simulink model "LKAS_AutoSave_DF_20220215_0920"  (R2018b)
settings: Solver=FixedStepDiscrete  StartTime=0.0  StopTime=10.0  FixedStep=0.01  RelTol=1e-3
InitFcn:
  | tmpVer = ver('MATLAB');
  | tmpVer = str2num(tmpVer.Version);
  | % -------------------------------------------------------------------
  | %  MATLAB file generated by Simulink.saveVars on 21-Nov-2019 10:06:14
  | %  MATLAB version: 7.13.0.564 (R2011b)
  | % -------------------------------------------------------------------
  | 
  | 
  | SInt16 = Simulink.AliasType;
  | SInt16.Description = 'Num';
  | if (tmpVer > 7.11)
  | 	SInt16.DataScope = 'Auto';
  | end
  | SInt16.HeaderFile = 'Rte_Type.h';
  | SInt16.BaseType = 'int16';
  | 
  | SInt32 = Simulink.AliasType;
  | SInt32.Description = 'Num';
  | if (tmpVer > 7.11)
  | 	SInt32.DataScope = 'Auto';
  | end
  | SInt32.HeaderFile = 'Rte_Type.h';
  | SInt32.BaseType = 'int32';
  | 
  | SInt8 = Simulink.AliasType;
  | SInt8.Description = 'Num';
  | if (tmpVer > 7.11)
  | 	SInt8.DataScope = 'Auto';
  | end
  | SInt8.HeaderFile = 'Rte_Type.h';
  | SInt8.BaseType = 'int8';
  | 
  | T_A_m2_1024_1_u32 = Simulink.NumericType;
  | T_A_m2_1024_1_u32.Description = 'm2 (square meters  (m2))';
  | if (tmpVer > 7.11)
  | 	T_A_m2_1024_1_u32.DataScope = 'Auto';
  | end
  | T_A_m2_1024_1_u32.HeaderFile = 'Rte_Type.h';
  | T_A_m2_1024_1_u32.DataTypeMode = 'Fixed-point: slope and bias scaling';
  | T_A_m2_1024_1_u32.SignednessBool = false;
  | T_A_m2_1024_1_u32.WordLength = 32;
  | T_A_m2_1024_1_u32.FixedExponent = -10;
  | T_A_m2_1024_1_u32.SlopeAdjustmentFactor = 1;
  | T_A_m2_1024_1_u32.Bias = 0;
  | T_A_m2_1024_1_u32.DataTypeOverride = 'Inherit';
  | T_A_m2_1024_1_u32.IsAlias = true;
  | 
  | T_A_m2_65536_1_u16 = Simulink.NumericType;
  | T_A_m2_65536_1_u16.Description = 'm2 (square meters  (m2))';
  | if (tmpVer > 7.11)
  | 	T_A_m2_65536_1_u16.DataScope = 'Auto';
  | end
  | T_A_m2_65536_1_u16.HeaderFile = 'Rte_Type.h';
  | T_A_m2_65536_1_u16.DataTypeMode = 'Fixed-point: slope and bias scaling';
  | T_A_m2_65536_1_u16.SignednessBool = false;
  | T_A_m2_65536_1_u16.WordLength = 16;
  | T_A_m2_65536_1_u16.FixedExponent = -16;
  | T_A_m2_65536_1_u16.SlopeAdjustmentFactor = 1;
  | T_A_m2_65536_1_u16.Bias = 0;
  | T_A_m2_65536_1_u16.DataTypeOverride = 'Inherit';
  | ... (+4647 lines)
StopFcn:
  | clear  T_A_m2_1024_1_u32 T_A_m2_65536_1_u16 T_A_m2_Float32 T_A_mm2_10_1_u16 T_A_mm2_4_1_s16 T_A_mm2_Float32 T_Cnt_Num_10_1_u32 T_Cnt_Num_1_1_s16 T_Cnt_Num_1_1_s32 T_Cnt_Num_1_1_s8 T_Cnt_Num_1_1_u16 T_Cnt_Num_1_1_u32 T_Cnt_Num_1_1_u8 T_E_J_1_1_s32 T_E_J_Float32 T_E_kJ_128_1_s32 T_E_kJ_Float32 T_E_kwh_10_1_u16 T_E_kwh_Float32 T_Epl_kwhpkm_100_1_u16 T_Epl_kwhpkm_Float32 T_F_N_1_1_s16 T_F_N_Float32 T_I_A_1000_1_u16 T_I_A_1048576_1_s32 T_I_A_2048_1_s16 T_I_A_32_1_s16 T_I_A_Float32 T_I_mA_1_1_s16 T_I_mA_32768_128_s16 T_I_mA_Float32 T_J_kgpm2_128_1_u16 T_J_kgpm2_Float32 T_K_NA_1000_1_s16 T_K_NA_100_1_s16 T_K_NA_100_1_u16 T_K_NA_1024_1_s16 T_K_NA_1024_1_u16 T_K_NA_128_1_s16 T_K_NA_128_1_u16 T_K_NA_128_1_u8 T_K_NA_16777216_1_u32 T_K_NA_16_1_s16 T_K_NA_16_1_u16 T_K_NA_16_1_u8 T_K_NA_1_16_u16 T_K_NA_1_1_s16 T_K_NA_1_1_u16 T_K_NA_1_1_u8 T_K_NA_32768_1_s16 T_K_NA_32768_1_u16 T_K_NA_32_1_s8 T_K_NA_4096_1_u16 T_K_NA_4194304_1_s32 T_K_NA_4194304_1_u16 T_K_NA_65536_1_s32 T_K_NA_65536_1_u16 T_K_NA_8192_1_s16 T_K_NA_8_1_s16 T_K_NA_Float32 T_M_Nm_16_1_s16 T_M_Nm_1_1_s16 T_M_Nm_32768_1_s16 T_M_Nm_32_1_s16 T_M_Nm_4_1_s16 T_M_Nm_512_1_s16 T_M_Nm_Float32 T_P_W_1_4_s16 T_P_W_1_8_s16 T_P_W_Float32 T_P_kW_128_1_s16 T_P_kW_1_8_s16 T_P_kW_8_1_s32 T_P_kW_Float32 T_Pct_pct_1024_1_s32 T_Pct_pct_1024_1_u32 T_Pct_pct_10_1_s16 T_Pct_pct_10_1_u32 T_Pct_pct_128_100_s8 T_Pct_pct_1_1_s16 T_Pct_pct_1_4_u8 T_Pct_pct_255_100_u16 T_Pct_pct_255_100_u8 T_Pct_pct_256_1_s16 T_Pct_pct_256_1_u16 T_Pct_pct_65535_100_u16 T_Pct_pct_Float32 T_R_ohm_1024_1_s16 T_R_ohm_32_1_s16 T_R_ohm_Float32 T_TK_K_16_1_s16 T_TK_K_Float32 T_T_degC_10_400_1_u16 T_T_degC_16_1_s16 T_T_degC_1_40_1_u8 T_T_degC_2_80_1_u8 T_T_degC_Float32 T_U_V_1000_1_u16 T_U_V_10_1_u8 T_U_V_200_1_u8 T_U_V_32_1_s16 T_U_V_4096_1_s16 T_U_V_512_1_s16 T_U_V_65535_8_u16 T_U_V_8192_1_u16 T_U_V_Float32 T_U_mV_1_1_s16 T_U_mV_256_20_u16 T_U_mV_Float32 T_V_l_256_1_s16 T_V_l_4096_1_s16 T_V_l_64_1_s16 T_V_l_65535_100_u16 T_V_l_Float32 T_V_ml_128_1_s16 T_V_ml_1_1_s16 T_V_ml_32768_1_s16 T_V_ml_Float32 T_V_ul_32_1_u16 T_V_ul_Float32 T_Vpl_clpkm_512_1_u16 T_Vpl_clpkm_Float32 T_a_kphps_16_1_s16 T_a_kphps_Float32 T_a_mps2_128_1_s16 T_a_mps2_Float32 T_c_MJpkg_256_1_s16 T_c_MJpkg_Float32 T_c_kJpgpK_1024_1_s16 T_c_kJpgpK_Float32 T_c_kJpkgpK_128_1_u16 T_c_kJpkgpK_Float32 T_chrg_Ah_1_1_s16 T_chrg_Ah_1_1_u16 T_chrg_Ah_1_1_u8 T_chrg_Ah_256_1_u16 T_chrg_Ah_4194304_1_s32 T_chrg_Ah_512_1_u16 T_chrg_Ah_8_1_u16 T_chrg_Ah_Float32 T_cmp_NA_100_1_s16 T_cmp_NA_128_1_s16 T_cmp_NA_16_1_s16 T_cmp_NA_32768_1_u16 T_cmp_NA_Float32 T_d2n_rpmps2_4_1_s16 T_d2n_rpmps2_Float32 T_dPct_pctps_16_1_s16 T_dPct_pctps_256_1_s16 T_dPct_pctps_Float32 T_dT_degCps_128_1_s16 T_dT_degCps_Float32 T_dV_lph_1_1_s16 T_dV_lph_Float32 T_dV_lpm_128_1_s16 T_dV_lpm_32_1_s16 T_dV_lpm_Float32 T_dV_lps_1024_1_u16 T_dV_lps_4_1_u16 T_dV_lps_Float32 T_dV_mlps_1024_1_s16 T_dV_mlps_Float32 T_d_BitField16 T_dm_gps_128_1_s16 T_dm_gps_128_1_u16 T_dm_gps_256_1_u16 T_dm_gps_Float32 T_dm_mgps_1_1_s16 T_dm_mgps_Float32 T_dn_rpmps_1_1_s16 T_dn_rpmps_2_1_s16 T_dn_rpmps_Float32 T_dp_Paps_1_1_s16 T_dp_Paps_Float32 T_dp_kPaps_1_1_s16 T_dp_kPaps_8_1_s16 T_dp_kPaps_Float32 T_dphi_degps_128_1_s16 T_dphi_degps_8_1_s16 T_dphi_degps_Float32 T_dr_ps_256_1_s16 T_dr_ps_Float32 T_drho_mgplps_1_2_s16 T_drho_mgplps_Float32 T_e_NA_1_1_u8 T_f_Hz_1_1_u16 T_f_Hz_1_1_u32 T_f_Hz_64_1_u16 T_f_Hz_8_1_s16 T_f_Hz_Float32 T_g_BitField32 T_l_km_16_1_s16 T_l_km_1_1_u16 T_l_km_1_1_u32 T_l_km_Float32 T_l_m_1024_1_s16 T_l_m_16_1_s16 T_l_m_1_1_u32 T_l_m_Float32 T_l_mm_16_1_s16 T_l_mm_1_1_u16 T_l_mm_4096_1_s16 T_l_mm_4_1_u8 T_l_mm_64_1_s16 T_l_mm_Float32 T_m_g_1_1_s16 T_m_g_2048_1_s16 T_m_g_32_1_u16 T_m_g_Float32 T_m_kg_1024_1_s16 T_m_kg_1_1_s16 T_m_kg_1_1_u32 T_m_kg_Float32 T_m_mg_128_1_s16 T_m_mg_32_1_s16 T_m_mg_Float32 T_n_rpm_1_1_s16 T_n_rpm_1_25_u8 T_n_rpm_256_50_u16 T_n_rpm_2_25_u8 T_n_rpm_4_1_u16 T_n_rpm_Float32 T_p_MPa_64_1_s16 T_p_MPa_Float32 T_p_Pa_1_1_s16 T_p_Pa_Float32 T_p_kPa_1_10_u16 T_p_kPa_1_1_s16 T_p_kPa_1_1_u8 T_p_kPa_256_1_u16 T_p_kPa_32_1_u16 T_p_kPa_64_1_s16 T_p_kPa_Float32 T_phi_deg_100_1_s16 T_phi_deg_1024_1_s16 T_phi_deg_128_1_s16 T_phi_deg_1_1_u8 T_phi_deg_256_1_s16 T_phi_deg_2_1_s8 T_phi_deg_32_1_s16 T_phi_deg_512_6_s32 T_phi_deg_Float32 T_phi_rad_2048_1_s16 T_phi_rad_Float32 T_r_NA_1024_1_s16 T_r_NA_1024_1_u16 T_r_NA_16384_1_s16 T_r_NA_16_1_s16 T_r_NA_256_1_s8 T_r_NA_256_1_u16 T_r_NA_32768_1_u16 T_r_NA_32_1_u16 T_r_NA_4096_1_s16 T_r_NA_65535_2_u16 T_r_NA_8192_1_u16 T_r_NA_Float32 T_rho_gpl_8192_1_s16 T_rho_gpl_Float32 T_rho_kgpm3_16_1_s16 T_rho_kgpm3_Float32 T_rho_mgpl_1_1_s16 T_rho_mgpl_64_1_s16 T_rho_mgpl_Float32 T_t_hour_1_1_s16 T_t_hour_Float32 T_t_m_1_1_u16 T_t_m_Float32 T_t_ms_1_1_s16 T_t_ms_1_1_u16 T_t_ms_1_1_u32 T_t_ms_4096_1_s16 T_t_ms_64_1_s16 T_t_ms_Float32 T_t_s_1000_1_s16 T_t_s_100_1_s16 T_t_s_10_1_s16 T_t_s_10_1_u16 T_t_s_1_1_s16 T_t_s_1_1_u16 T_t_s_1_1_u32 T_t_s_Float32 T_t_us_10_1_u32 T_t_us_1_1_s16 T_t_us_1_1_u32 T_t_us_1_4_u16 T_t_us_Float32 T_v_kph_1_1_u8 T_v_kph_64_1_s16 T_v_kph_64_1_u16 T_v_kph_Float32 T_v_mps_256_1_s16 T_v_mps_Float32 T_w_radps_32_1_s16 T_w_radps_Float32 T_y_BitField8 T_y_BitFieldDiagProgress T_y_BitFieldDiagStatus T_y_NA_1_1_u8 SInt16 SInt32 SInt8 T_BOOLEAN UInt16 UInt32 UInt8 s16 s32 s8 u16 u32 u8
model workspace (MAT data in the model file):
  MCOS : class17 (value not decoded)
  MCOS : class17 (value not decoded)
  MCOS : class17 (value not decoded)
  MCOS : class17 (value not decoded)
  MCOS : class17 (value not decoded)
  MCOS : class17 (value not decoded)
  MCOS : class17 (value not decoded)
  MCOS : class17 (value not decoded)
  MCOS : class17 (value not decoded)
  MCOS : class17 (value not decoded)
  MCOS : class17 (value not decoded)
  MCOS : class17 (value not decoded)
  MCOS : class17 (value not decoded)
  MCOS : class17 (value not decoded)
  MCOS : class17 (value not decoded)
  MCOS : class17 (value not decoded)
  MCOS : class17 (value not decoded)
  MCOS : class17 (value not decoded)
  MCOS : class17 (value not decoded)
  MCOS : class17 (value not decoded)
  MCOS : class17 (value not decoded)
  MCOS : class17 (value not decoded)
  MCOS : class17 (value not decoded)
  MCOS : class17 (value not decoded)
  MCOS : class17 (value not decoded)
  MCOS : class17 (value not decoded)
  MCOS : class17 (value not decoded)
  MCOS : class17 (value not decoded)
  MCOS : class17 (value not decoded)
  MCOS : class17 (value not decoded)
  MCOS : class17 (value not decoded)
  MCOS : class17 (value not decoded)
  MCOS : class17 (value not decoded)
  MCOS : class17 (value not decoded)
  MCOS : class17 (value not decoded)
  MCOS : class17 (value not decoded)
  MCOS : class17 (value not decoded)
  MCOS : class17 (value not decoded)
  MCOS : class17 (value not decoded)
  MCOS : class17 (value not decoded)
  MCOS : class17 (value not decoded)
  MCOS : class17 (value not decoded)
  MCOS : class17 (value not decoded)
  MCOS : class17 (value not decoded)
  MCOS : class17 (value not decoded)
  MCOS : class17 (value not decoded)
  MCOS : class17 (value not decoded)
  MCOS : class17 (value not decoded)
  MCOS : class17 (value not decoded)
  MCOS : class17 (value not decoded)
  MCOS : class17 (value not decoded)
  MCOS : class17 (value not decoded)
  MCOS : class17 (value not decoded)
  MCOS : class17 (value not decoded)
  MCOS : class17 (value not decoded)
  MCOS : class17 (value not decoded)
  MCOS : class17 (value not decoded)
  MCOS : class17 (value not decoded)
  MCOS : class17 (value not decoded)
  MCOS : class17 (value not decoded)
  MCOS : class17 (value not decoded)
  MCOS : class17 (value not decoded)
  MCOS : class17 (value not decoded)
  MCOS : class17 (value not decoded)
  MCOS : class17 (value not decoded)
  MCOS : class17 (value not decoded)
  MCOS : class17 (value not decoded)
  MCOS : class17 (value not decoded)
  MCOS : class17 (value not decoded)
  MCOS : class17 (value not decoded)
  MCOS : class17 (value not decoded)
  MCOS : class17 (value not decoded)
  MCOS : class17 (value not decoded)
  MCOS : class17 (value not decoded)
  MCOS : class17 (value not decoded)
  MCOS : class17 (value not decoded)
  MCOS : class17 (value not decoded)
  MCOS : class17 (value not decoded)
  MCOS : class17 (value not decoded)
  MCOS : class17 (value not decoded)
  MCOS : class17 (value not decoded)
  MCOS : class17 (value not decoded)
  MCOS : class17 (value not decoded)
  MCOS : class17 (value not decoded)
  MCOS : class17 (value not decoded)
  MCOS : class17 (value not decoded)
  MCOS : class17 (value not decoded)
  MCOS : class17 (value not decoded)
  MCOS : class17 (value not decoded)
  MCOS : class17 (value not decoded)
  MCOS : class17 (value not decoded)
  MCOS : class17 (value not decoded)
  MCOS : class17 (value not decoded)
  MCOS : class17 (value not decoded)
  MCOS : class17 (value not decoded)
  MCOS : class17 (value not decoded)
  MCOS : class17 (value not decoded)
  MCOS : class17 (value not decoded)
  MCOS : class17 (value not decoded)
  MCOS : class17 (value not decoded)
  MCOS : class17 (value not decoded)
  MCOS : class17 (value not decoded)
undefined symbols (not defined in the file): LKA_CarWidth, LKA_SampleTime, LKA_StrRatio_C, LKA_Veh2CamL_C, LKA_Veh2CamW_C, LKA_WhlBaseL_C, LL_CompHdAg_C, LL_CompSWA_C, LL_CrvtPrvwT_C, LL_DesDvt_C, LL_DvtComp_C, LL_DvtPrvwT_C, LL_DvtSpdDet_vDvtSpdMin_C, LL_HandsOff_ExitTime, LL_HandsOff_TextTime, LL_HandsOff_WarnTime, LL_HdAgExT_C, LL_HdAgPrvwT_C, LL_LAccMax_C, LL_LAccRMax_C, LL_LDW_EarliestWarnLine_C, LL_LDW_LatestWarnLine_C, LL_LDWS_SUPPRESS_HEADING, LL_LFClb_TFC_FfCtlRatio_C, LL_LFClb_TFC_KdBalance_C, LL_LFClb_TFC_KdMaxSWA_C, LL_LFClb_TFC_KdV1_C, LL_LFClb_TFC_KdV2_C, LL_LFClb_TFC_KdVehSpdLwr_C, LL_LFClb_TFC_KdVehSpdUpr_C, LL_LFClb_TFC_Ki_C, LL_LFClb_TFC_KiMaxSWA_C, LL_LFClb_TFC_Kp_C, LL_LFClb_TFC_KpKlat_C, LL_LFClb_TFC_KpV1_C, LL_LFClb_TFC_KpV2_C, LL_LFClb_TFC_KpVehSpdLwr_C, LL_LFClb_TFC_KpVehSpdUpr_C, LL_LFClb_TFC_PrvwT_C, LL_LKA_EarliestWarnLine_C, LL_LKA_LatestWarnLine_C, LL_LKAExPrcs_ExitC0Dvt, LL_LKAExPrcs_ExitC0Swt, LL_LKAExPrcs_tiExitTime1, LL_LKAExPrcs_tiExitTime2, LL_LKAExPrcs_tiExitTime3, LL_LKAS_OUT_OF_CONTROL_LAT_VEL, LL_LKAS_OUT_OF_CONTROL_TTLC, LL_LKASWASyn_M0, LL_LKASWASyn_M1, LL_LKASWASyn_M2, LL_LKASWASyn_M3K, LL_LKASWASyn_SWAaddMax, LL_LKASWASyn_T2, LL_LKASWASyn_tiTrqSwaRtTime, LL_LKASWASyn_tiTrqSwaTime, LL_LKASWASyn_TrqMax, LL_LKASWASyn_TrqSwaAddSwt, LL_LKASWASyn_TrqSwaRateDiff, LL_LSpdCompT_C ... (+43)
libraries: simulink x136, canmsglib x8, dspstat3 x3, simulink_extras x1
(part 4 of 20)

== system LKAS_AutoSave_DF_20220215_0920/LKAS/Monitor ==
  CAN Pack : canmsglib/CAN Pack  MsgList=(none)  MsgName=CAN Msg  MsgIDType=Standard (11-bit identifier)  MsgIdentifier=1  MsgLength=8  SignalInfo=Signal1$8$16$2$2$1$0$0.01$0$-Inf$Inf$#Signal2$24$16$2$2$1$0$0.01$0$-Inf$Inf$#Signal3$40$16$2$2$1$0$0.01$0$-Inf$Inf$#Signal4$56$16$2$2$1$0$0.01$0$-Inf$Inf$#  NSignals=4  StartBits=str2num('[int32(8);int32(24);int32(40);int32(56)]')  SignalSizes=str2num('[int32(16);int32(16);int32(16);int32(16)]')  ByteOrders=str2num('[int32(2);int32(2);int32(2);int32(2)]')  DataTypes=str2num('[int32(2);int32(2);int32(2);int32(2)]')  MultiplexTypes=str2num('[int32(1);int32(1);int32(1);int32(1)]')  MultiplexValues=str2num('[double(0);double(0);double(0);double(0)]')  Factors=str2num('[double(0.01);double(0.01);double(0.01);double(0.01)]')  Offsets=str2num('[double(0);double(0);double(0);double(0)]')  Minimums=str2num('[double(-Inf);double(-Inf);double(-Inf);double(-Inf)]')  Maximums=str2num('[double(Inf);double(Inf);double(Inf);double(Inf)]')  Remote=off  ApplyMinMax=off  BusOutput=on
      settings: SourceProductName=Simulink Real-Time  SourceProductBaseCode=XP  DataFormat=manually specified signals
  CAN Pack1 : canmsglib/CAN Pack  MsgList=(none)  MsgName=CAN Msg  MsgIDType=Standard (11-bit identifier)  MsgIdentifier=2  MsgLength=8  SignalInfo=Signal1$8$16$2$2$1$0$0.01$0$-Inf$Inf$#Signal2$24$16$2$2$1$0$0.01$0$-Inf$Inf$#Signal3$40$16$2$2$1$0$0.01$0$-Inf$Inf$#Signal4$56$16$2$2$1$0$0.01$0$-Inf$Inf$#  NSignals=4  StartBits=str2num('[int32(8);int32(24);int32(40);int32(56)]')  SignalSizes=str2num('[int32(16);int32(16);int32(16);int32(16)]')  ByteOrders=str2num('[int32(2);int32(2);int32(2);int32(2)]')  DataTypes=str2num('[int32(2);int32(2);int32(2);int32(2)]')  MultiplexTypes=str2num('[int32(1);int32(1);int32(1);int32(1)]')  MultiplexValues=str2num('[double(0);double(0);double(0);double(0)]')  Factors=str2num('[double(0.01);double(0.01);double(0.01);double(0.01)]')  Offsets=str2num('[double(0);double(0);double(0);double(0)]')  Minimums=str2num('[double(-Inf);double(-Inf);double(-Inf);double(-Inf)]')  Maximums=str2num('[double(Inf);double(Inf);double(Inf);double(Inf)]')  Remote=off  ApplyMinMax=off  BusOutput=on
      settings: SourceProductName=Simulink Real-Time  SourceProductBaseCode=XP  DataFormat=manually specified signals
  CAN Pack2 : canmsglib/CAN Pack  MsgList=(none)  MsgName=CAN Msg  MsgIDType=Standard (11-bit identifier)  MsgIdentifier=3  MsgLength=8  SignalInfo=Signal1$8$16$2$2$1$0$0.01$0$-Inf$Inf$#Signal2$24$16$2$2$1$0$0.01$0$-Inf$Inf$#Signal3$40$16$2$2$1$0$0.01$0$-Inf$Inf$#Signal4$56$16$2$2$1$0$0.01$0$-Inf$Inf$#  NSignals=4  StartBits=str2num('[int32(8);int32(24);int32(40);int32(56)]')  SignalSizes=str2num('[int32(16);int32(16);int32(16);int32(16)]')  ByteOrders=str2num('[int32(2);int32(2);int32(2);int32(2)]')  DataTypes=str2num('[int32(2);int32(2);int32(2);int32(2)]')  MultiplexTypes=str2num('[int32(1);int32(1);int32(1);int32(1)]')  MultiplexValues=str2num('[double(0);double(0);double(0);double(0)]')  Factors=str2num('[double(0.01);double(0.01);double(0.01);double(0.01)]')  Offsets=str2num('[double(0);double(0);double(0);double(0)]')  Minimums=str2num('[double(-Inf);double(-Inf);double(-Inf);double(-Inf)]')  Maximums=str2num('[double(Inf);double(Inf);double(Inf);double(Inf)]')  Remote=off  ApplyMinMax=off  BusOutput=on
      settings: SourceProductName=Simulink Real-Time  SourceProductBaseCode=XP  DataFormat=manually specified signals
  CAN Pack3 : canmsglib/CAN Pack  MsgList=(none)  MsgName=CAN Msg  MsgIDType=Standard (11-bit identifier)  MsgIdentifier=4  MsgLength=8  SignalInfo=Signal1$8$16$2$2$1$0$0.01$0$-Inf$Inf$#Signal2$24$16$2$2$1$0$0.01$0$-Inf$Inf$#Signal3$40$16$2$2$1$0$0.01$0$-Inf$Inf$#Signal4$56$16$2$2$1$0$0.01$0$-Inf$Inf$#  NSignals=4  StartBits=str2num('[int32(8);int32(24);int32(40);int32(56)]')  SignalSizes=str2num('[int32(16);int32(16);int32(16);int32(16)]')  ByteOrders=str2num('[int32(2);int32(2);int32(2);int32(2)]')  DataTypes=str2num('[int32(2);int32(2);int32(2);int32(2)]')  MultiplexTypes=str2num('[int32(1);int32(1);int32(1);int32(1)]')  MultiplexValues=str2num('[double(0);double(0);double(0);double(0)]')  Factors=str2num('[double(0.01);double(0.01);double(0.01);double(0.01)]')  Offsets=str2num('[double(0);double(0);double(0);double(0)]')  Minimums=str2num('[double(-Inf);double(-Inf);double(-Inf);double(-Inf)]')  Maximums=str2num('[double(Inf);double(Inf);double(Inf);double(Inf)]')  Remote=off  ApplyMinMax=off  BusOutput=on
      settings: SourceProductName=Simulink Real-Time  SourceProductBaseCode=XP  DataFormat=manually specified signals
  CAN Unpack : canmsglib/CAN Unpack  MsgList=(none)  MsgName=CAN Msg  MsgIDType=Standard (11-bit identifier)  MsgIdentifier=1  MsgLength=8  SignalInfo=Signal1$24$32$2$2$1$0$1$0$-Inf$Inf$#Signal2$56$32$2$2$1$0$1$0$-Inf$Inf$#  NSignals=2  IDPort=off  TimestampPort=off  ErrorPort=off  RemotePort=off  LengthPort=off  StatusPort=off  StartBits=str2num('[int32(24);int32(56)]')  SignalSizes=str2num('[int32(32);int32(32)]')  ByteOrders=str2num('[int32(2);int32(2)]')  DataTypes=str2num('[int32(2);int32(2)]')  MultiplexTypes=str2num('[int32(1);int32(1)]')  MultiplexValues=str2num('[double(0);double(0)]')  Factors=str2num('[double(1);double(1)]')  Offsets=str2num('[double(0);double(0)]')  Minimums=str2num('[double(-Inf);double(-Inf)]')  Maximums=str2num('[double(Inf);double(Inf)]')  ApplyMinMax=off
      settings: SourceProductName=Simulink Real-Time  SourceProductBaseCode=XP
  CAN Unpack1 : canmsglib/CAN Unpack  MsgList=(none)  MsgName=CAN Msg  MsgIDType=Standard (11-bit identifier)  MsgIdentifier=2  MsgLength=8  SignalInfo=Signal1$24$32$2$2$1$0$1$0$-Inf$Inf$#Signal2$56$32$2$2$1$0$1$0$-Inf$Inf$#  NSignals=2  IDPort=off  TimestampPort=off  ErrorPort=off  RemotePort=off  LengthPort=off  StatusPort=off  StartBits=str2num('[int32(24);int32(56)]')  SignalSizes=str2num('[int32(32);int32(32)]')  ByteOrders=str2num('[int32(2);int32(2)]')  DataTypes=str2num('[int32(2);int32(2)]')  MultiplexTypes=str2num('[int32(1);int32(1)]')  MultiplexValues=str2num('[double(0);double(0)]')  Factors=str2num('[double(1);double(1)]')  Offsets=str2num('[double(0);double(0)]')  Minimums=str2num('[double(-Inf);double(-Inf)]')  Maximums=str2num('[double(Inf);double(Inf)]')  ApplyMinMax=off
      settings: SourceProductName=Simulink Real-Time  SourceProductBaseCode=XP
  CAN Unpack2 : canmsglib/CAN Unpack  MsgList=(none)  MsgName=CAN Msg  MsgIDType=Standard (11-bit identifier)  MsgIdentifier=3  MsgLength=8  SignalInfo=Signal1$24$32$2$2$1$0$1$0$-Inf$Inf$#Signal2$56$32$2$2$1$0$1$0$-Inf$Inf$#  NSignals=2  IDPort=off  TimestampPort=off  ErrorPort=off  RemotePort=off  LengthPort=off  StatusPort=off  StartBits=str2num('[int32(24);int32(56)]')  SignalSizes=str2num('[int32(32);int32(32)]')  ByteOrders=str2num('[int32(2);int32(2)]')  DataTypes=str2num('[int32(2);int32(2)]')  MultiplexTypes=str2num('[int32(1);int32(1)]')  MultiplexValues=str2num('[double(0);double(0)]')  Factors=str2num('[double(1);double(1)]')  Offsets=str2num('[double(0);double(0)]')  Minimums=str2num('[double(-Inf);double(-Inf)]')  Maximums=str2num('[double(Inf);double(Inf)]')  ApplyMinMax=off
      settings: SourceProductName=Simulink Real-Time  SourceProductBaseCode=XP
  CAN Unpack3 : canmsglib/CAN Unpack  MsgList=(none)  MsgName=CAN Msg  MsgIDType=Standard (11-bit identifier)  MsgIdentifier=4  MsgLength=8  SignalInfo=Signal1$24$32$2$2$1$0$1$0$-Inf$Inf$#Signal2$56$32$2$2$1$0$1$0$-Inf$Inf$#  NSignals=2  IDPort=off  TimestampPort=off  ErrorPort=off  RemotePort=off  LengthPort=off  StatusPort=off  StartBits=str2num('[int32(24);int32(56)]')  SignalSizes=str2num('[int32(32);int32(32)]')  ByteOrders=str2num('[int32(2);int32(2)]')  DataTypes=str2num('[int32(2);int32(2)]')  MultiplexTypes=str2num('[int32(1);int32(1)]')  MultiplexValues=str2num('[double(0);double(0)]')  Factors=str2num('[double(1);double(1)]')  Offsets=str2num('[double(0);double(0)]')  Minimums=str2num('[double(-Inf);double(-Inf)]')  Maximums=str2num('[double(Inf);double(Inf)]')  ApplyMinMax=off
      settings: SourceProductName=Simulink Real-Time  SourceProductBaseCode=XP
  Cast To Single{1..10,21..26} (16 alike) : DataTypeConversion  OutDataTypeStr=single
  LLBus : BusSelector  OutputSignals=InPMon.LFTTTLC_Mon,InPMon.RGTTTLC_Mon,StateMon.LDW_State_Mon,StateMon.LKA_State_Mon,LKAMon.LKA_ExitFlg_Mon,LKAMon.LKA_SampleTime_Mon,LKAMon.T1_Mon,Disable_Reason
  LKASve_g_ob5H_10 : Outport  OutDataTypeStr=UInt32
  LKASve_g_ob5L_10 : Outport  Port=2  OutDataTypeStr=UInt32
  LKASve_g_ob6H_10 : Outport  Port=3  OutDataTypeStr=UInt32
  LKASve_g_ob6L_10 : Outport  Port=4  OutDataTypeStr=UInt32
  LKASve_g_ob07H_100 : Outport  Port=5  OutDataTypeStr=UInt32
  LKASve_g_ob07L_100 : Outport  Port=6  OutDataTypeStr=UInt32
  LKASve_g_ob08H_100 : Outport  Port=7  OutDataTypeStr=UInt32
  LKASve_g_ob08L_100 : Outport  Port=8  OutDataTypeStr=UInt32
  wires:
  LLBus/5 -> [LKA_ExitFlg_Mon]  "<LKA_ExitFlg_Mon>"
  LLBus/6 -> [LKA_SampleTime_Mon]  "<LKA_SampleTime_Mon>"
  LLBus/3 -> [LDW_State_Mon]  "<LDW_State_Mon>"
  LLBus/7 -> [T1_Mon]  "<T1_Mon>"
  LLBus/4 -> [LKA_State_Mon]  "<LKA_State_Mon>"
  LLBus/2 -> [RGTTTLC_Mon]  "<RGTTTLC_Mon>"
  LLBus/1 -> [LFTTTLC_Mon]  "<LFTTTLC_Mon>"
  [LLMon] -> LLBus/1
  [LKA_State_Mon] -> Cast To Single4/1
  [LDW_State_Mon] -> Cast To Single3/1
  CAN Pack/1 -> CAN Unpack/1
  CAN Unpack/1 -> LKASve_g_ob5H_10/1  "LKASve_g_ob5H_10"
  CAN Unpack/2 -> LKASve_g_ob5L_10/1  "LKASve_g_ob5L_10"
  CAN Pack1/1 -> CAN Unpack1/1
  [LKA_ExitFlg_Mon] -> Cast To Single5/1
  [LKA_SampleTime_Mon] -> Cast To Single6/1
  [T1_Mon] -> Cast To Single7/1
  [Disable_Reason] -> Cast To Single8/1
  CAN Unpack1/1 -> LKASve_g_ob6H_10/1  "LKASve_g_ob6H_10"
  CAN Unpack1/2 -> LKASve_g_ob6L_10/1  "LKASve_g_ob6L_10"
  CAN Pack2/1 -> CAN Unpack2/1
  [Monitor9] -> Cast To Single9/1
  [Monitor10] -> Cast To Single10/1
  [Monitor11] -> Cast To Single21/1
  [Monitor12] -> Cast To Single22/1
  CAN Unpack2/1 -> LKASve_g_ob07H_100/1  "LKASve_g_ob07H_100"
  CAN Unpack2/2 -> LKASve_g_ob07L_100/1  "LKASve_g_ob07L_100"
  CAN Pack3/1 -> CAN Unpack3/1
  CAN Unpack3/2 -> LKASve_g_ob08L_100/1  "LKASve_g_ob08L_100"
  CAN Unpack3/1 -> LKASve_g_ob08H_100/1  "LKASve_g_ob08H_100"
  [Monitor15] -> Cast To Single24/1
  [Monitor14] -> Cast To Single23/1
  [Monitor13] -> Cast To Single26/1
  [Monitor16] -> Cast To Single25/1
  Cast To Single1/1 -> CAN Pack/1
  Cast To Single2/1 -> CAN Pack/2
  Cast To Single3/1 -> CAN Pack/3
  Cast To Single4/1 -> CAN Pack/4
  Cast To Single5/1 -> CAN Pack1/1
  Cast To Single6/1 -> CAN Pack1/2
  Cast To Single7/1 -> CAN Pack1/3
  Cast To Single8/1 -> CAN Pack1/4
  Cast To Single22/1 -> CAN Pack2/4
  Cast To Single10/1 -> CAN Pack2/2
  Cast To Single21/1 -> CAN Pack2/3
  Cast To Single9/1 -> CAN Pack2/1
  Cast To Single24/1 -> CAN Pack3/3
  Cast To Single23/1 -> CAN Pack3/2
  Cast To Single25/1 -> CAN Pack3/4
  Cast To Single26/1 -> CAN Pack3/1
  [LFTTTLC_Mon] -> Cast To Single1/1
  [RGTTTLC_Mon] -> Cast To Single2/1
  LLBus/8 -> [Disable_Reason]  "<Disable_Reason>"

== system LKAS_AutoSave_DF_20220215_0920/LKAS/Output ==
  bsLLOut : Inport
  Bus Selector : BusSelector  OutputSignals=Vehicle_Lane_Display,LDW_Status_Display,LKA_Status_Display,LDW_Flag,Hands_Off_Warning,LKA_Action_Indication,HMI_Popup_Status,LKA_Torque_Req,LKA_TorqueReq_Value,EPS_State_Ctl,LKA_SWA_Control,EPS_Factor_Control,EPS_LKA_Control
  Cast To Single{1..9,12} (10 alike) : DataTypeConversion  OutDataTypeStr=UInt8
  Cast To Single10 : DataTypeConversion  OutDataTypeStr=T_M_Nm_Float32
  Cast To Single11 : DataTypeConversion  OutDataTypeStr=T_M_Nm_Float32
  Cast To Single13 : DataTypeConversion  OutDataTypeStr=T_M_Nm_Float32
  Vehicle_Lane_Display : Outport
  LDW_Status_Display : Outport  Port=2
  LKA_Status_Display : Outport  Port=3
  LDW_Flag : Outport  Port=4
  Hands_Off_Warning : Outport  Port=5
  LKA_Action_Indication : Outport  Port=6
  HMI_Popup_Status : Outport  Port=7
  LKA_TorqueReq : Outport  Port=8
  LKA_TorqueReq_Value : Outport  Port=9
  EPS_State_Control : Outport  Port=10
  LKA_SWA_Control : Outport  Port=11
  EPS_Factor_Control : Outport  Port=12
  EPS_LKA_Control : Outport  Port=13
  wires:
  Cast To Single1/1 -> Vehicle_Lane_Display/1  "Vehicle_Lane_Display"
  Cast To Single2/1 -> LDW_Status_Display/1  "LDW_Status_Display"
  Cast To Single3/1 -> LKA_Status_Display/1  "LKA_Status_Display"
  Cast To Single4/1 -> LDW_Flag/1  "LDW_Flag"
  Cast To Single5/1 -> Hands_Off_Warning/1  "Hands_Off_Warning"
  Cast To Single6/1 -> LKA_Action_Indication/1  "LKA_Action_Indication"
  Cast To Single7/1 -> HMI_Popup_Status/1  "HMI_Popup_Status"
  Cast To Single8/1 -> EPS_State_Control/1  "EPS_State_Control"
  Cast To Single9/1 -> EPS_LKA_Control/1  "EPS_LKA_Control"
  Cast To Single10/1 -> EPS_Factor_Control/1  "EPS_Factor_Control"
  Cast To Single11/1 -> LKA_SWA_Control/1  "LKA_SWA_Control"
  Cast To Single12/1 -> LKA_TorqueReq/1  "LKA_TorqueReq"
  Cast To Single13/1 -> LKA_TorqueReq_Value/1  "LKA_TorqueReq_Value"
  Bus Selector/9 -> Cast To Single13/1  "<LKA_TorqueReq_Value>"
  Bus Selector/8 -> Cast To Single12/1  "<LKA_Torque_Req>"
  Bus Selector/4 -> Cast To Single4/1  "<LDW_Flag>"
  Bus Selector/3 -> Cast To Single3/1  "<LKA_Status_Display>"
  Bus Selector/12 -> Cast To Single10/1  "<EPS_Factor_Control>"
  Bus Selector/6 -> Cast To Single6/1  "<LKA_Action_Indication>"
  Bus Selector/7 -> Cast To Single7/1  "<HMI_Popup_Status>"
  Bus Selector/5 -> Cast To Single5/1  "<Hands_Off_Warning>"
  Bus Selector/1 -> Cast To Single1/1  "<Vehicle_Lane_Display>"
  Bus Selector/10 -> Cast To Single8/1  "<EPS_State_Ctl>"
  bsLLOut/1 -> Bus Selector/1  "bsLLOutput"
  Bus Selector/11 -> Cast To Single11/1  "<LKA_SWA_Control>"
  Bus Selector/13 -> Cast To Single9/1  "<EPS_LKA_Control>"
  Bus Selector/2 -> Cast To Single2/1  "<LDW_Status_Display>"

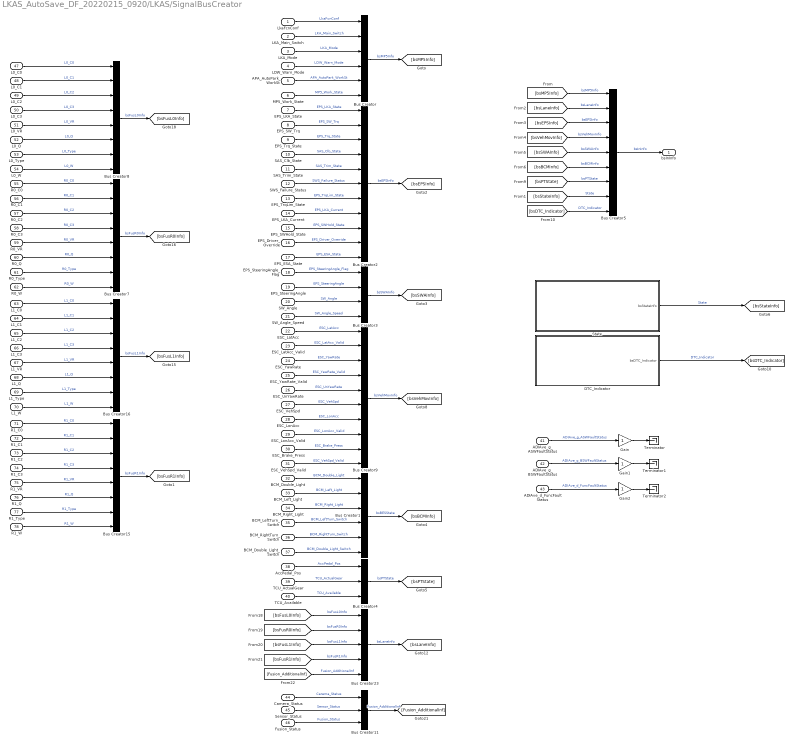
== system LKAS_AutoSave_DF_20220215_0920/LKAS/SignalBusCreator ==
  LkaFcnConf : Inport
  LKA_Main_Switch : Inport  Port=2
  LKA_Mode : Inport  Port=3
  LDW_Warn_Mode : Inport  Port=4
  APA_AutoPark_WorkSt : Inport  Port=5
  MP5_Work_State : Inport  Port=6
  EPS_LKA_State : Inport  Port=7
  EPS_SW_Trq : Inport  Port=8
  EPS_Trq_State : Inport  Port=9
  SAS_Clb_State : Inport  Port=10
  SAS_Trim_State : Inport  Port=11
  SWS_Failure_Status : Inport  Port=12
  EPS_TrqLim_State : Inport  Port=13
  EPS_LKA_Current : Inport  Port=14
  EPS_SWHold_State : Inport  Port=15
  EPS_Driver_Override : Inport  Port=16
  EPS_ESA_State : Inport  Port=17
  EPS_SteeringAngle_Flag : Inport  Port=18
  EPS_SteeringAngle : Inport  Port=19
  SW_Angle : Inport  Port=20
  SW_Angle_Speed : Inport  Port=21
  ESC_LatAcc : Inport  Port=22
  ESC_LatAcc_Valid : Inport  Port=23
  ESC_YawRate : Inport  Port=24
  ESC_YawRate_Valid : Inport  Port=25
  ESC_UnYawRate : Inport  Port=26
  ESC_VehSpd : Inport  Port=27
  ESC_LonAcc : Inport  Port=28
  ESC_LonAcc_Valid : Inport  Port=29
  ESC_Brake_Press : Inport  Port=30
  ESC_VehSpd_Valid : Inport  Port=31
  BCM_Double_Light : Inport  Port=32
  BCM_Left_Light : Inport  Port=33
  BCM_Right_Light : Inport  Port=34
  BCM_LeftTurn_Switch : Inport  Port=35
  BCM_RightTurn_Switch : Inport  Port=36
  BCM_Double_Light_Switch : Inport  Port=37
  AccPedal_Pos : Inport  Port=38
  TCU_ActualGear : Inport  Port=39
  TCU_Available : Inport  Port=40
  ADIAve_g_ASWFaultStatus : Inport  Port=41
  ADIAve_g_BSWFaultStatus : Inport  Port=42
  ADIAve_d_FuncFaultStatus : Inport  Port=43
  Camera_Status : Inport  Port=44
  Sensor_Status : Inport  Port=45
  Fusion_Status : Inport  Port=46
  L0_C0 : Inport  Port=47
  L0_C1 : Inport  Port=48
  L0_C2 : Inport  Port=49
  L0_C3 : Inport  Port=50
  L0_VR : Inport  Port=51
  L0_Q : Inport  Port=52
  L0_Type : Inport  Port=53
  L0_W : Inport  Port=54
  R0_C0 : Inport  Port=55
  R0_C1 : Inport  Port=56
  R0_C2 : Inport  Port=57
  R0_C3 : Inport  Port=58
  R0_VR : Inport  Port=59
  R0_Q : Inport  Port=60
  R0_Type : Inport  Port=61
  R0_W : Inport  Port=62
  L1_C0 : Inport  Port=63
  L1_C1 : Inport  Port=64
  L1_C2 : Inport  Port=65
  L1_C3 : Inport  Port=66
  L1_VR : Inport  Port=67
  L1_Q : Inport  Port=68
  L1_Type : Inport  Port=69
  L1_W : Inport  Port=70
  R1_C0 : Inport  Port=71
  R1_C1 : Inport  Port=72
  R1_C2 : Inport  Port=73
  R1_C3 : Inport  Port=74
  R1_VR : Inport  Port=75
  R1_Q : Inport  Port=76
  R1_Type : Inport  Port=77
  R1_W : Inport  Port=78
  Bus Creator : BusCreator  Inputs=6
  Bus Creator1 : BusCreator  Inputs=6
  Bus Creator11 : BusCreator  Inputs=3
  Bus Creator{7..8,15..16} (4 alike) : BusCreator  Inputs=8
  Bus Creator2 : BusCreator  Inputs=11
  Bus Creator23 : BusCreator  Inputs=5
  Bus Creator3 : BusCreator  Inputs=4
  Bus Creator4 : BusCreator  Inputs=3
  Bus Creator5 : BusCreator  Inputs=9
  Bus Creator9 : BusCreator  Inputs=10
  DTC_Indicator : Subsystem
  Gain : Gain
  Gain1 : Gain
  Gain2 : Gain
  State : Subsystem
  Terminator : Terminator
  Terminator1 : Terminator
  Terminator2 : Terminator
  bsInInfo : Outport
  wires:
  Bus Creator9/1 -> [bsVehMovInfo]  "bsVehMovInfo"
  Bus Creator3/1 -> [bsSWAInfo]  "bsSWAInfo"
  Bus Creator1/1 -> [bsBCMInfo]  "bsBESState"
  Bus Creator2/1 -> [bsEPSInfo]  "bsEPSInfo"
  Bus Creator/1 -> [bsMP5Info]  "bsMP5Info"
  [bsLaneInfo] -> Bus Creator5/2  "bsLaneInfo"
  [bsEPSInfo] -> Bus Creator5/3  "bsEPSInfo"
  [bsVehMovInfo] -> Bus Creator5/4  "bsVehMovInfo"
  [bsSWAInfo] -> Bus Creator5/5  "bsSWAInfo"
  [bsBCMInfo] -> Bus Creator5/6  "bsBCMInfo"
  [bsPTState] -> Bus Creator5/7  "bsPTState"
  [bsMP5Info] -> Bus Creator5/1  "bsMP5Info"
  [bsStateInfo] -> Bus Creator5/8  "State"
  [bsDTC_Indicator] -> Bus Creator5/9  "DTC_Indicator"
  Bus Creator4/1 -> [bsPTState]  "bsPTState"
  Bus Creator7/1 -> [bsFusR0Info]  "bsFusR0Info"
  Bus Creator16/1 -> [bsFusL1Info]  "bsFusL1Info"
  Bus Creator15/1 -> [bsFusR1Info]  "bsFusR1Info"
  Bus Creator8/1 -> [bsFusL0Info]  "bsFusL0Info"
  [bsFusL0Info] -> Bus Creator23/1  "bsFusL0Info"
  [bsFusR0Info] -> Bus Creator23/2  "bsFusR0Info"
  [bsFusL1Info] -> Bus Creator23/3  "bsFusL1Info"
  [bsFusR1Info] -> Bus Creator23/4  "bsFusR1Info"
  Bus Creator23/1 -> [bsLaneInfo]  "bsLaneInfo"
  [Fusion_AdditionalInf] -> Bus Creator23/5  "Fusion_AdditionalInf"
  DTC_Indicator/1(bsDTC_Indicator) -> [bsDTC_Indicator]  "DTC_Indicator"
  State/1(bsStateInfo) -> [bsStateInfo]  "State"
  Bus Creator5/1 -> bsInInfo/1  "bsInInfo"
  AccPedal_Pos/1 -> Bus Creator4/1  "AccPedal_Pos"
  TCU_ActualGear/1 -> Bus Creator4/2  "TCU_ActualGear"
  BCM_Double_Light/1 -> Bus Creator1/1  "BCM_Double_Light"
  BCM_Left_Light/1 -> Bus Creator1/2  "BCM_Left_Light"
  BCM_Right_Light/1 -> Bus Creator1/3  "BCM_Right_Light"
  SW_Angle/1 -> Bus Creator3/3  "SW_Angle"
  SW_Angle_Speed/1 -> Bus Creator3/4  "SW_Angle_Speed"
  SWS_Failure_Status/1 -> Bus Creator2/6  "SWS_Failure_Status"
  ESC_LatAcc/1 -> Bus Creator9/1  "ESC_LatAcc"
  ESC_LatAcc_Valid/1 -> Bus Creator9/2  "ESC_LatAcc_Valid"
  ESC_YawRate/1 -> Bus Creator9/3  "ESC_YawRate"
  ESC_YawRate_Valid/1 -> Bus Creator9/4  "ESC_YawRate_Valid"
  ESC_UnYawRate/1 -> Bus Creator9/5  "ESC_UnYawRate"
  ESC_VehSpd/1 -> Bus Creator9/6  "ESC_VehSpd"
  ESC_LonAcc/1 -> Bus Creator9/7  "ESC_LonAcc"
  ESC_LonAcc_Valid/1 -> Bus Creator9/8  "ESC_LonAcc_Valid"
  ESC_Brake_Press/1 -> Bus Creator9/9  "ESC_Brake_Press"
  ESC_VehSpd_Valid/1 -> Bus Creator9/10  "ESC_VehSpd_Valid"
  EPS_LKA_State/1 -> Bus Creator2/1  "EPS_LKA_State"
  EPS_SW_Trq/1 -> Bus Creator2/2  "EPS_SW_Trq"
  EPS_Trq_State/1 -> Bus Creator2/3  "EPS_Trq_State"
  SAS_Clb_State/1 -> Bus Creator2/4  "SAS_Clb_State"
  SAS_Trim_State/1 -> Bus Creator2/5  "SAS_Trim_State"
  EPS_TrqLim_State/1 -> Bus Creator2/7  "EPS_TrqLim_State"
  EPS_LKA_Current/1 -> Bus Creator2/8  "EPS_LKA_Current"
  EPS_SWHold_State/1 -> Bus Creator2/9  "EPS_SWHold_State"
  LKA_Main_Switch/1 -> Bus Creator/2  "LKA_Main_Switch"
  LKA_Mode/1 -> Bus Creator/3  "LKA_Mode"
  L0_C0/1 -> Bus Creator8/1  "L0_C0"
  L0_C1/1 -> Bus Creator8/2  "L0_C1"
  L0_C2/1 -> Bus Creator8/3  "L0_C2"
  L0_C3/1 -> Bus Creator8/4  "L0_C3"
  L0_VR/1 -> Bus Creator8/5  "L0_VR"
  L0_Q/1 -> Bus Creator8/6  "L0_Q"
  L0_Type/1 -> Bus Creator8/7  "L0_Type"
  L0_W/1 -> Bus Creator8/8  "L0_W"
  R0_C0/1 -> Bus Creator7/1  "R0_C0"
  R0_C1/1 -> Bus Creator7/2  "R0_C1"
  R0_C2/1 -> Bus Creator7/3  "R0_C2"
  R0_C3/1 -> Bus Creator7/4  "R0_C3"
  R0_VR/1 -> Bus Creator7/5  "R0_VR"
  R0_Q/1 -> Bus Creator7/6  "R0_Q"
  R0_Type/1 -> Bus Creator7/7  "R0_Type"
  R0_W/1 -> Bus Creator7/8  "R0_W"
  L1_C0/1 -> Bus Creator16/1  "L1_C0"
  L1_C1/1 -> Bus Creator16/2  "L1_C1"
  L1_C2/1 -> Bus Creator16/3  "L1_C2"
  L1_C3/1 -> Bus Creator16/4  "L1_C3"
  L1_VR/1 -> Bus Creator16/5  "L1_VR"
  L1_Q/1 -> Bus Creator16/6  "L1_Q"
  L1_Type/1 -> Bus Creator16/7  "L1_Type"
  L1_W/1 -> Bus Creator16/8  "L1_W"
  R1_C0/1 -> Bus Creator15/1  "R1_C0"
  R1_C1/1 -> Bus Creator15/2  "R1_C1"
  R1_C2/1 -> Bus Creator15/3  "R1_C2"
  R1_C3/1 -> Bus Creator15/4  "R1_C3"
  R1_VR/1 -> Bus Creator15/5  "R1_VR"
  R1_Q/1 -> Bus Creator15/6  "R1_Q"
  R1_Type/1 -> Bus Creator15/7  "R1_Type"
  R1_W/1 -> Bus Creator15/8  "R1_W"
  TCU_Available/1 -> Bus Creator4/3  "TCU_Available"
  BCM_LeftTurn_Switch/1 -> Bus Creator1/4  "BCM_LeftTurn_Switch"
  BCM_RightTurn_Switch/1 -> Bus Creator1/5  "BCM_RightTurn_Switch"
  EPS_SteeringAngle_Flag/1 -> Bus Creator3/1  "EPS_SteeringAngle_Flag"
  EPS_SteeringAngle/1 -> Bus Creator3/2  "EPS_SteeringAngle"
  EPS_Driver_Override/1 -> Bus Creator2/10  "EPS_Driver_Override"
  Bus Creator11/1 -> [Fusion_AdditionalInf]  "Fusion_AdditionalInf"
  Camera_Status/1 -> Bus Creator11/1  "Carema_Status"
  Sensor_Status/1 -> Bus Creator11/2  "Sensor_Status"
  Fusion_Status/1 -> Bus Creator11/3  "Fusion_Status"
  MP5_Work_State/1 -> Bus Creator/6  "MP5_Work_State"
  APA_AutoPark_WorkSt/1 -> Bus Creator/5  "APA_AutoPark_WorkSt"
  LDW_Warn_Mode/1 -> Bus Creator/4  "LDW_Warn_Mode"
  LkaFcnConf/1 -> Bus Creator/1  "LkaFcnConf"
  EPS_ESA_State/1 -> Bus Creator2/11  "EPS_ESA_State"
  ADIAve_g_ASWFaultStatus/1 -> Gain/1  "ADIAve_g_ASWFaultStatus"
  Gain/1 -> Terminator/1
  Gain1/1 -> Terminator1/1
  ADIAve_g_BSWFaultStatus/1 -> Gain1/1  "ADIAve_g_BSWFaultStatus"
  Gain2/1 -> Terminator2/1
  ADIAve_d_FuncFaultStatus/1 -> Gain2/1  "ADIAve_d_FuncFaultStatus"
  BCM_Double_Light_Switch/1 -> Bus Creator1/6  "BCM_Double_Light_Switch"

== system LKAS_AutoSave_DF_20220215_0920/LKAS/LL/Fault_Diagnostic ==
  bsInInfo : Inport
  Bus Creator : BusCreator  Inputs=2
  Bus Creator1 : BusCreator  Inputs=10
  Bus Selector3 : BusSelector  OutputSignals=DTC_Indicator.LKAS_BSWDTC_Status
  Bus Selector4 : BusSelector  OutputSignals=bsVehMovInfo.ESC_VehSpd_Valid,bsEPSInfo.EPS_LKA_State,bsEPSInfo.SAS_Clb_State,bsEPSInfo.SAS_Trim_State,bsPTState.TCU_ActualGear,bsEPSInfo.EPS_TrqLim_State,bsEPSInfo.EPS_Trq_State,bsVehMovInfo.ESC_LatAcc_Valid,bsVehMovInfo.ESC_YawRate_Valid,bsVehMovInfo.ESC_LonAcc_Valid
  Compare To Constant26 : simulink/Logic and Bit Operations/Compare To Constant  relop=~=  const=1  OutDataTypeStr=boolean
  Compare To Constant27 : simulink/Logic and Bit Operations/Compare To Constant  relop===  const=4  OutDataTypeStr=boolean
  Compare To Constant29 : simulink/Logic and Bit Operations/Compare To Constant  relop===  const=0  OutDataTypeStr=boolean
  Compare To Constant{30,36..39} (5 alike) : simulink/Logic and Bit Operations/Compare To Constant  relop===  const=1  OutDataTypeStr=boolean
  Compare To Constant34 : simulink/Logic and Bit Operations/Compare To Constant  relop=>  const=3  OutDataTypeStr=boolean
  Compare To Constant35 : simulink/Logic and Bit Operations/Compare To Constant  relop===  const=0  OutDataTypeStr=boolean
  bsSignalFault : Outport
  wires:
  Bus Creator/1 -> bsSignalFault/1
  Bus Selector3/1 -> Bus Creator/1  "<LKAS_BSWDTC_Status>"
  bsInInfo/1 -> Bus Selector4/1, Bus Selector3/1
  Bus Selector4/1 -> Compare To Constant26/1  "<ESC_VehSpd_Valid>"
  Compare To Constant26/1 -> Bus Creator1/1  "Event_FaulVehSpeed"
  Bus Selector4/2 -> Compare To Constant27/1  "<EPS_LKA_State>"
  Bus Selector4/3 -> Compare To Constant29/1  "<SAS_Clb_State>"
  Compare To Constant29/1 -> Bus Creator1/3  "Event_FaulSASClb"
  Bus Selector4/4 -> Compare To Constant30/1  "<SAS_Trim_State>"
  Bus Selector4/5 -> Compare To Constant34/1  "<TCU_ActualGear>"
  Bus Selector4/6 -> Compare To Constant35/1  "<EPS_TrqLim_State>"
  Bus Selector4/7 -> Compare To Constant36/1  "<EPS_Trq_State>"
  Bus Selector4/8 -> Compare To Constant37/1  "<ESC_LatAcc_Valid>"
  Bus Selector4/9 -> Compare To Constant38/1  "<ESC_YawRate_Valid>"
  Bus Selector4/10 -> Compare To Constant39/1  "<ESC_LonAcc_Valid>"
  Compare To Constant30/1 -> Bus Creator1/4  "Event_FaulSASTrim"
  Compare To Constant35/1 -> Bus Creator1/6  "Event_FaulTrqLim"
  Compare To Constant34/1 -> Bus Creator1/5  "Event_FaulTCUGear"
  Compare To Constant36/1 -> Bus Creator1/7  "Event_FaulEPSTrqSt"
  Compare To Constant37/1 -> Bus Creator1/8  "Event_FaulLatAcc"
  Compare To Constant38/1 -> Bus Creator1/9  "Event_FaulYawRate"
  Compare To Constant39/1 -> Bus Creator1/10  "Event_FaulLonAcc"
  Bus Creator1/1 -> Bus Creator/2  "LKAS_ASWDTC_Status"
  Compare To Constant27/1 -> Bus Creator1/2  "Event_FaulEPSLKASt"

== system LKAS_AutoSave_DF_20220215_0920/LKAS/LL/Human Machine Interface (HMI) ==
  HMI_stDACmode : Inport
  HMI_LKA_STATE : Inport  Port=2
  HMI_LDW_STATE : Inport  Port=3
  HMI_LDWWarn : Inport  Port=4
  HMI_R0_Quality : Inport  Port=5
  HMI_L0_Quality : Inport  Port=6
  HMI_EPSInfo : Inport  Port=7
  HMI_camera_common_fault : Inport  Port=8
  HMI_Front_Camera_Blocked : Inport  Port=9
  HMI_bsLLClb : Inport  Port=10
  Bus Creator2 : BusCreator  Inputs=7
  Bus Selector : BusSelector  OutputSignals=bsConstantClb.LKA_SampleTime,bsLLSMConClb.DisblCClb.LL_HandsOff_TextTime,bsLLSMConClb.DisblCClb.LL_HandsOff_WarnTime
  Cast To Single{,1..6} (7 alike) : DataTypeConversion  OutDataTypeStr=uint8
  Ground : Ground
  HMI_Popup_Status : MATLAB Function  TreatAsAtomicUnit=on
  Hands_Off_Warning : MATLAB Function  TreatAsAtomicUnit=on
  LDW_Flag : MATLAB Function  TreatAsAtomicUnit=on
  LDW_Status_Display : MATLAB Function  TreatAsAtomicUnit=on
  LKA_Status_Display : MATLAB Function  TreatAsAtomicUnit=on
  LKA_action_indication : MATLAB Function  TreatAsAtomicUnit=on
  Subsystem : Subsystem
  Vehicle_Lane_Display : MATLAB Function  TreatAsAtomicUnit=on
  HMI_LDWLKA : Outport
  wires:
  Bus Creator2/1 -> HMI_LDWLKA/1
  Hands_Off_Warning/1(Hands_Off_Warning) -> Cast To Single4/1  "Hands_Off_Warning"
  Cast To Single5/1 -> Bus Creator2/6  "LKA_Action_Indication"
  Cast To Single2/1 -> Bus Creator2/3  "LKA_Status_Display"
  LDW_Flag/1(LDW_Flag) -> Cast To Single3/1  "LDW_Flag"
  LDW_Status_Display/1(LDW_Status_Display) -> Cast To Single1/1  "LDW_Status_Display"
  HMI_Popup_Status/1(HMI_Popup_Status) -> Cast To Single6/1  "HMI_Popup_Status"
  Cast To Single1/1 -> Bus Creator2/2  "LDW_Status_Display"
  LKA_Status_Display/1(LKA_Status_Display) -> Cast To Single2/1  "LKA_Status_Display"
  Cast To Single3/1 -> Bus Creator2/4  "LDW_Flag"
  Vehicle_Lane_Display/1(Vehicle_Lane_Display) -> Cast To Single/1  "Vehicle_Lane_Display"
  Cast To Single/1 -> Bus Creator2/1  "Vehicle_Lane_Display"
  Cast To Single6/1 -> Bus Creator2/7  "HMI_Popup_Status"
  LKA_action_indication/1(LKA_Action_Indication) -> Cast To Single5/1  "LKA_Action_Indication"
  Cast To Single4/1 -> Bus Creator2/5  "Hands_Off_Warning"
  HMI_LKA_STATE/1 -> Vehicle_Lane_Display/2(LKA_STATE), LKA_action_indication/2(LKA_STATE), HMI_Popup_Status/2(LKA_STATE), LDW_Flag/2(HMI_LKA_STATE), LKA_Status_Display/2(LKA_STATE), Subsystem/2(LKA_STATE)  "HMI_LKA_STATE"
  HMI_LDW_STATE/1 -> Vehicle_Lane_Display/3(LDW_STATE), LDW_Status_Display/2(LDW_STATE), Subsystem/1(LDW_STATE)  "HMI_LDW_STATE"
  Ground/1 -> HMI_Popup_Status/6(stFaultCSyn)  "HMI_stFaultCSyn"
  HMI_L0_Quality/1 -> Vehicle_Lane_Display/5(L0_Quality)  "HMI_L0_Quality"
  HMI_stDACmode/1 -> Vehicle_Lane_Display/1(stDACmode), LDW_Status_Display/1(stDACmode), LKA_action_indication/1(stDACmode), HMI_Popup_Status/1(stDACmode), LDW_Flag/1(HMI_stDACmode), LKA_Status_Display/1(stDACmode)  "HMI_stDACmode"
  HMI_Front_Camera_Blocked/1 -> HMI_Popup_Status/5(Front_Camera_Blocked)  "HMI_Front_Camera_Blocked"
  HMI_R0_Quality/1 -> Vehicle_Lane_Display/4(R0_Quality)  "HMI_R0_Quality"
  HMI_camera_common_fault/1 -> HMI_Popup_Status/4(camera_common_fault)  "HMI_camera_common_fault"
  HMI_EPSInfo/1 -> Subsystem/3(EPSInfo)  "HMI_EPSInfo"
  Subsystem/2(HandsOff1_Text) -> HMI_Popup_Status/3(HandsOff)
  Subsystem/1(HandsOff2_Warn) -> Hands_Off_Warning/1(HandsOff)
  HMI_LDWWarn/1 -> LDW_Flag/3(HMI_LDWWarnInfo)
  HMI_bsLLClb/1 -> Bus Selector/1  "HMI_bsLLClb"
  Bus Selector/1 -> Subsystem/4(SampleTime)  "<LKA_SampleTime>"
  Bus Selector/2 -> Subsystem/5(HandsOff_Text)  "<LL_HandsOff_TextTime>"
  Bus Selector/3 -> Subsystem/6(HandsOff_Warn)  "<LL_HandsOff_WarnTime>"

== system LKAS_AutoSave_DF_20220215_0920/LKAS/LL/LL Inputs Mapping ==
  bsInInfo : Inport
  bsLLClb : Inport  Port=2
  Bus Creator : BusCreator  Inputs=7
  Bus Selector : BusSelector  OutputSignals=bsMP5Info,bsLaneInfo,bsEPSInfo,bsVehMovInfo,bsSWAInfo,bsBCMInfo,bsPTState
  bsBCMInfo : Subsystem
  bsEPSInfo : Subsystem
  bsLaneInfo : Subsystem
  bsMP5Info : Subsystem
  bsPTState : Subsystem
  bsSWAInfo : Subsystem
  bsVehMovInfo : Subsystem
  bsInfo : Outport
  wires:
  bsSWAInfo/1(bsSWAInfoOut) -> Bus Creator/5  "bsSWAInfo"
  bsLaneInfo/1(bsLaneInfoOut) -> Bus Creator/2  "bsLaneInfo"
  bsPTState/1(bsPTStateOut) -> Bus Creator/7  "bsPTState"
  Bus Selector/7 -> bsPTState/1(bsPTStateIn)  "<bsPTState>"
  bsBCMInfo/1(bsBCMInfoOut) -> Bus Creator/6  "bsBCMInfo"
  bsMP5Info/1(bsMP5InfoOut) -> Bus Creator/1  "bsMP5Info"
  Bus Selector/1 -> bsMP5Info/1(bsMP5InfoIn)  "<bsMP5Info>"
  Bus Selector/6 -> bsBCMInfo/1(bsBCMInfoIn)  "<bsBCMInfo>"
  Bus Selector/5 -> bsSWAInfo/1(bsSWAInfoIn)  "<bsSWAInfo>"
  bsVehMovInfo/1(bsVehMovInfoOut) -> Bus Creator/4  "bsVehMovInfo"
  Bus Selector/4 -> bsVehMovInfo/1(bsVehMovInfoIn)  "<bsVehMovInfo>"
  bsEPSInfo/1(bsEPSInfoOut) -> Bus Creator/3  "bsEPSInfo"
  Bus Selector/3 -> bsEPSInfo/1(bsEPSInfoIn)  "<bsEPSInfo>"
  Bus Selector/2 -> bsLaneInfo/2(bsLaneInfoIn)  "<bsLaneInfo>"
  Bus Creator/1 -> bsInfo/1
  bsInInfo/1 -> Bus Selector/1
  bsLLClb/1 -> bsLaneInfo/1(bsLLClb)

== system LKAS_AutoSave_DF_20220215_0920/LKAS/LL/LLOn ==
  bsInInfo : Inport
  bsLLClb : Inport  Port=2
  bsSignalFault : Inport  Port=3
  Enable : EnablePort  StatesWhenEnabling=reset
      settings: AttributesFormatString=states = %<StatesWhenEnabling>
  LDW : Subsystem  Description=|  TreatAsAtomicUnit=on
      | Block Name: Lane Departure Warning
      | Ab.: LDW
      | No.: 1.3.0.0
      | Rev: 0.0.1
      | Update Date: 19-3-26
  LKA : Subsystem  Description=|  TreatAsAtomicUnit=on
      | Block Name: Lane Keeping Assistance
      | Ab.: LKA
      | No.: 1.2.0.0
      | Rev: 0.0.1
      | Update Date: 19-5-13
  LKA Input Processing (LKAInP) : Subsystem
  LL State Determination (LLStateDet) : Subsystem
  LL_Mon : Subsystem
  bsLLState : Outport  OutputWhenDisabled=reset  InitialOutput=0
      settings: AttributesFormatString=%<OutputWhenDisabled> = %<InitialOutput>
  LDW_Flag : Outport  Port=2  OutputWhenDisabled=reset  InitialOutput=0
      settings: AttributesFormatString=%<OutputWhenDisabled> = %<InitialOutput>
  phiSWACmd : Outport  Port=3  OutputWhenDisabled=reset  InitialOutput=0
      settings: AttributesFormatString=%<OutputWhenDisabled> = %<InitialOutput>
  M : Outport  Port=4  OutputWhenDisabled=reset  InitialOutput=0
      settings: AttributesFormatString=%<OutputWhenDisabled> = %<InitialOutput>
  LLMon : Outport  Port=5
      settings: AttributesFormatString=%<OutputWhenDisabled> = %<InitialOutput>
  wires:
  LL State Determination (LLStateDet)/2(LLStateDet_stLDWActvFlg) -> LDW/Enable
  [bsLLClb] -> LL State Determination (LLStateDet)/3(LLStateDet_bsLLClb)
  [bsLLClb] -> LKA Input Processing (LKAInP)/2(LKAInP_bsLLClb)
  LL State Determination (LLStateDet)/1(LLStateDet_bsLLState) -> bsLLState/1
  [bsLLClb] -> LDW/2(LDW_bsLDWClb)
  LKA Input Processing (LKAInP)/1(LKAInP_bsLKAInPInfo) -> LL State Determination (LLStateDet)/2(LLStateDet_bsLKAInPInfo), LKA/2(LKA_bsLKAInPInfo)
  bsLLClb/1 -> [bsLLClb]
  LL State Determination (LLStateDet)/3(LLStateDet_stLKAActvFlg) -> LKA/Enable, [ActFlg]
  LDW/1(LDW_Flag) -> LDW_Flag/1  "LDW_Flag"
  bsInInfo/1 -> LKA/1(LKA_bsInInfoSyn), LDW/1(LDW_bsInInfoSyn), LL State Determination (LLStateDet)/1(LLStateDet_bsInInfoSyn), LKA Input Processing (LKAInP)/1(LKAInP_bsInInfoSyn)
  [ExitFlg] -> LL State Determination (LLStateDet)/4(LLStateDet_stExitFlg)
  LKA/2(LKA_phiSWACmd) -> phiSWACmd/1  "OutputSWACmd"
  LKA/1(LKA_ExitFlg) -> [ExitFlg]
  bsSignalFault/1 -> LL State Determination (LLStateDet)/5(LLStateDet_SignalFault)
  LKA/3(LKA_M) -> M/1  "OutputM"
  LKA/4(LKAMon) -> [LKAMon]
  [LKAMon] -> LL_Mon/2(LKAMon)
  LL_Mon/1(LLMon) -> LLMon/1
  [bsLLClb] -> LKA/3(LKA_bsLKAClb)
  [ActFlg] -> LKA Input Processing (LKAInP)/3(In3)
  LL State Determination (LLStateDet)/4(Disable_Reason) -> LL_Mon/1(Disable_Reason)
